simulink model "Cardiovascularmodel"  (Simulink 7.4)
settings: Solver=ode45  StartTime=0.0  StopTime=10.0  RelTol=1e-3
undefined symbols (not defined in the file): magnitude
(part 1 of 2)
settings Model: Creator=Marek  LastModifiedBy=Marek

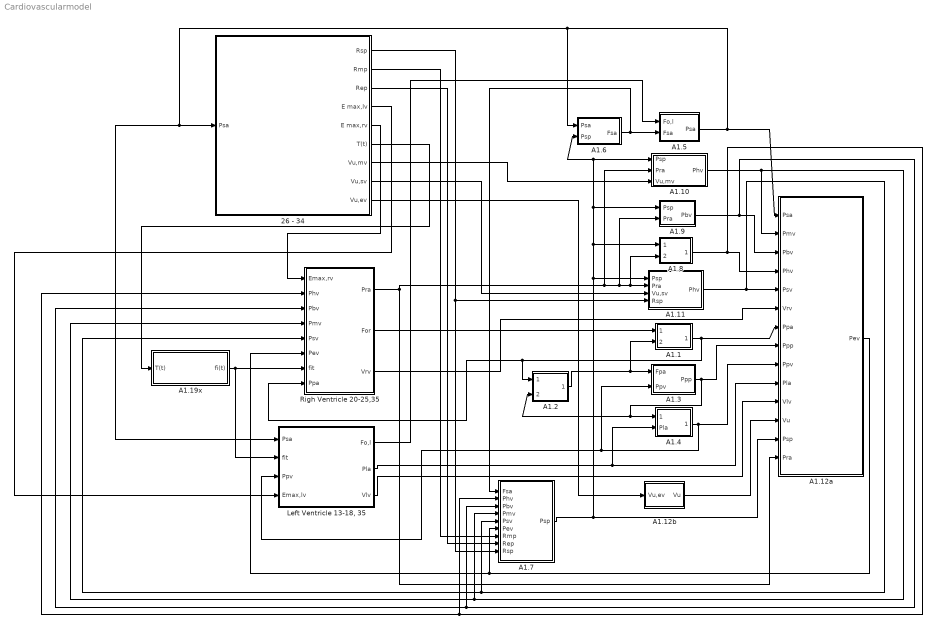
== system Cardiovascularmodel ==
  26 - 34 : Subsystem
  A1.1 : Subsystem
  A1.10 : Subsystem
  A1.11 : Subsystem
  A1.12a : Subsystem
  A1.12b : Subsystem
  A1.19x : Subsystem
  A1.2 : Subsystem
  A1.3 : Subsystem
  A1.4 : Subsystem
  A1.5 : Subsystem
  A1.6 : Subsystem
  A1.7 : Subsystem
  A1.8 : Subsystem
  A1.9 : Subsystem
  "Left Ventricle 13-18, 35" : Subsystem
  Righ Ventricle 20-25,35 : Subsystem
  wires:
  A1.11/1(Phv) -> A1.12a/5(Psv), A1.7/5(Psv), Righ Ventricle 20-25,35/5(Psv)
  A1.5/1(Psa) -> A1.12a/1(Psa), A1.6/1(Psa), 26 - 34/1(Psa), "Left Ventricle 13-18, 35"/1(Psa)
  A1.10/1(Phv) -> A1.12a/2(Pmv), A1.7/4(Pmv), Righ Ventricle 20-25,35/4(Pmv)
  A1.9/1(Pbv) -> A1.12a/3(Pbv), A1.7/3(Pbv), Righ Ventricle 20-25,35/3(Pbv)
  A1.8/1(Phv) -> A1.12a/4(Phv), A1.7/2(Phv), Righ Ventricle 20-25,35/2(Phv)
  Righ Ventricle 20-25,35/3(Vrv) -> A1.12a/6(Vrv)
  A1.1/1(Ppa) -> A1.12a/7(Ppa), A1.2/1(Ppa), Righ Ventricle 20-25,35/8(Ppa)
  A1.3/1(Ppp) -> A1.12a/8(Ppp), A1.2/2(Ppp), A1.4/1(Ppp)
  A1.4/1(Ppv) -> A1.12a/9(Ppv), A1.3/2(Ppv), "Left Ventricle 13-18, 35"/3(Ppv)
  "Left Ventricle 13-18, 35"/2(Pla) -> A1.12a/10(Pla), A1.4/2(Pla)
  A1.12b/1(Vu) -> A1.12a/12(Vu)
  A1.7/1(Psp) -> A1.12a/13(Psp), A1.8/1(Psp), A1.10/1(Psp), A1.6/2(Psp), A1.9/1(Psp), A1.11/1(Psp)
  A1.2/1(Fpa) -> A1.3/1(Fpa), A1.1/2(Fpa)
  Righ Ventricle 20-25,35/1(Pra) -> A1.12a/14(Pra), A1.11/2(Pra), A1.8/2(Pra), A1.9/2(Pra), A1.10/2(Pra)
  A1.6/1(Fsa) -> A1.5/2(Fsa), A1.7/1(Fsa)
  A1.19x/1(fi(t)) -> Righ Ventricle 20-25,35/7(fit), "Left Ventricle 13-18, 35"/2(fit)
  A1.12a/1(Pev) -> A1.7/6(Pev), Righ Ventricle 20-25,35/6(Pev)
  26 - 34/6(T(t)) -> A1.19x/1(T(t))
  "Left Ventricle 13-18, 35"/3(Vlv) -> A1.12a/11(Vlv)
  26 - 34/7(Vu,mv) -> A1.10/3(Vu,mv)
  26 - 34/8(Vu,sv) -> A1.11/3(Vu,sv)
  "Left Ventricle 13-18, 35"/1(Fo,l) -> A1.5/1(Fo,l)
  Righ Ventricle 20-25,35/2(For) -> A1.1/1(Fo,r)
  26 - 34/1(Rsp) -> A1.7/9(Rsp), A1.11/4(Rsp)
  26 - 34/2(Rmp) -> A1.7/7(Rmp)
  26 - 34/3(Rep) -> A1.7/8(Rep)
  26 - 34/9(Vu,ev) -> A1.12b/1(Vu,ev)
  26 - 34/5(E max,rv) -> Righ Ventricle 20-25,35/1(Emax,rv)
  26 - 34/4(E max,lv) -> "Left Ventricle 13-18, 35"/4(Emax,lv)

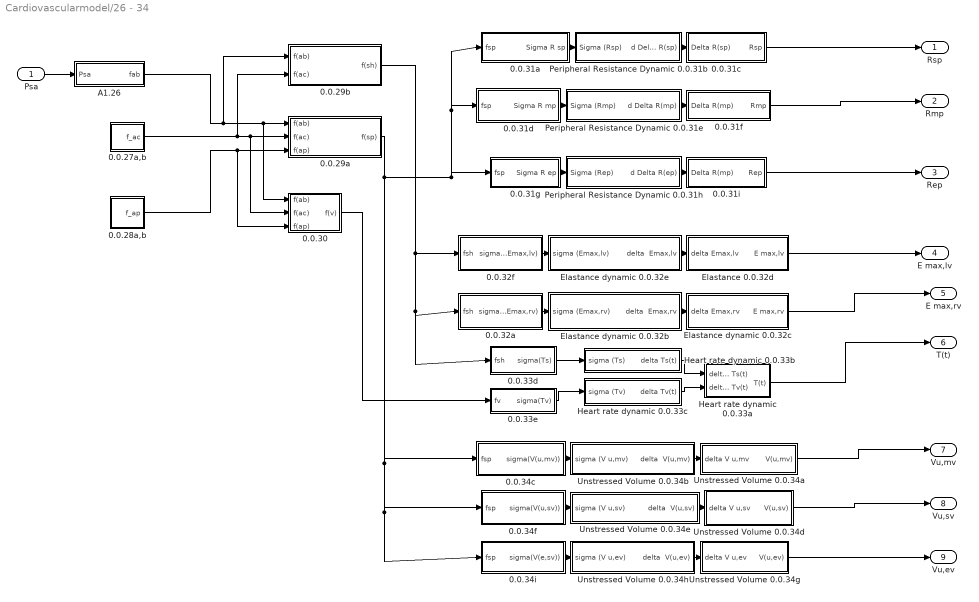
== system Cardiovascularmodel/26 - 34 ==
  Psa : Inport  OutDataType=fixdt(1, 16)  OutScaling=2^0
  0.0.27a,b : Subsystem
  0.0.28a,b : Subsystem
  0.0.29a : Subsystem
  0.0.29b : Subsystem
  0.0.30 : Subsystem
  0.0.31a : Subsystem
  0.0.31c : Subsystem
  0.0.31d : Subsystem
  0.0.31f : Subsystem
  0.0.31g : Subsystem
  0.0.31i : Subsystem
  0.0.32a : Subsystem
  0.0.32f : Subsystem
  0.0.33d : Subsystem
  0.0.33e : Subsystem
  0.0.34c : Subsystem
  0.0.34f : Subsystem
  0.0.34i : Subsystem
  A1.26 : Subsystem
  Elastance 0.0.32d : Subsystem
  Elastance dynamic 0.0.32b : Subsystem
  Elastance dynamic 0.0.32c : Subsystem
  Elastance dynamic 0.0.32e : Subsystem
  Heart rate dynamic 0.0.33a : Subsystem
  Heart rate dynamic 0.0.33b : Subsystem
  Heart rate dynamic 0.0.33c : Subsystem
  Peripheral Resistance Dynamic 0.0.31b : Subsystem
  Peripheral Resistance Dynamic 0.0.31e : Subsystem
  Peripheral Resistance Dynamic 0.0.31h : Subsystem
  Unstressed Volume 0.0.34a : Subsystem
  Unstressed Volume 0.0.34b : Subsystem
  Unstressed Volume 0.0.34d : Subsystem
  Unstressed Volume 0.0.34e : Subsystem
  Unstressed Volume 0.0.34g : Subsystem
  Unstressed Volume 0.0.34h : Subsystem
  Rsp : Outport  OutDataType=fixdt(1, 16)  OutScaling=2^0
  Rmp : Outport  Port=2  OutDataType=fixdt(1, 16)  OutScaling=2^0
  Rep : Outport  Port=3  OutDataType=fixdt(1, 16)  OutScaling=2^0
  E max,lv : Outport  Port=4  OutDataType=fixdt(1, 16)  OutScaling=2^0
  E max,rv : Outport  Port=5  OutDataType=fixdt(1, 16)  OutScaling=2^0
  T(t) : Outport  Port=6  OutDataType=fixdt(1, 16)  OutScaling=2^0
  Vu,mv : Outport  Port=7  OutDataType=fixdt(1, 16)  OutScaling=2^0
  Vu,sv : Outport  Port=8  OutDataType=fixdt(1, 16)  OutScaling=2^0
  Vu,ev : Outport  Port=9  OutDataType=fixdt(1, 16)  OutScaling=2^0
  wires:
  A1.26/1(fab) -> 0.0.29a/1(f(ab)), 0.0.30/1(f(ab)), 0.0.29b/1(f(ab))
  0.0.27a,b/1(f_ac) -> 0.0.29a/2(f(ac)), 0.0.30/2(f(ac)), 0.0.29b/2(f(ac))
  0.0.28a,b/1(f_ap) -> 0.0.29a/3(f(ap)), 0.0.30/3(f(ap))
  Elastance dynamic 0.0.32e/1(delta  Emax,lv) -> Elastance 0.0.32d/1(delta Emax,lv)
  0.0.32f/1(sigma(Emax,lv)) -> Elastance dynamic 0.0.32e/1(sigma (Emax,lv))
  Elastance dynamic 0.0.32b/1(delta  Emax,rv) -> Elastance dynamic 0.0.32c/1(delta Emax,rv)
  0.0.32a/1(sigma(Emax,rv)) -> Elastance dynamic 0.0.32b/1(sigma (Emax,rv))
  Heart rate dynamic 0.0.33c/1(delta Tv(t)) -> Heart rate dynamic 0.0.33a/2(delta Tv(t))
  0.0.33d/1(sigma(Ts)) -> Heart rate dynamic 0.0.33b/1(sigma (Ts))
  0.0.33e/1(sigma(Tv)) -> Heart rate dynamic 0.0.33c/1(sigma (Tv))
  Heart rate dynamic 0.0.33b/1(delta Ts(t)) -> Heart rate dynamic 0.0.33a/1(delta Ts(t))
  Unstressed Volume 0.0.34b/1(delta  V(u,mv)) -> Unstressed Volume 0.0.34a/1(delta V u,mv)
  0.0.34c/1(sigma(V(u,mv))) -> Unstressed Volume 0.0.34b/1(sigma (V u,mv))
  Unstressed Volume 0.0.34e/1(delta  V(u,sv)) -> Unstressed Volume 0.0.34d/1(delta V u,sv)
  0.0.34f/1(sigma(V(u,sv))) -> Unstressed Volume 0.0.34e/1(sigma (V u,sv))
  Unstressed Volume 0.0.34h/1(delta  V(u,ev)) -> Unstressed Volume 0.0.34g/1(delta V u,ev)
  0.0.34i/1(sigma(V(e,sv))) -> Unstressed Volume 0.0.34h/1(sigma (V u,ev))
  0.0.31a/1(Sigma R sp) -> Peripheral Resistance Dynamic 0.0.31b/1(Sigma (Rsp))
  Peripheral Resistance Dynamic 0.0.31b/1(d Delta R(sp)) -> 0.0.31c/1(Delta R(sp))
  0.0.31d/1(Sigma R mp) -> Peripheral Resistance Dynamic 0.0.31e/1(Sigma (Rmp))
  Peripheral Resistance Dynamic 0.0.31e/1(d Delta R(mp)) -> 0.0.31f/1(Delta R(mp))
  0.0.31g/1(Sigma R ep) -> Peripheral Resistance Dynamic 0.0.31h/1(Sigma (Rep))
  Peripheral Resistance Dynamic 0.0.31h/1(d Delta R(ep)) -> 0.0.31i/1(Delta R(mp))
  Psa/1 -> A1.26/1(Psa)
  0.0.29b/1(f(sh)) -> 0.0.32f/1(fsh), 0.0.32a/1(fsh), 0.0.33d/1(fsh)
  0.0.29a/1(f(sp)) -> 0.0.34i/1(fsp), 0.0.34f/1(fsp), 0.0.34c/1(fsp), 0.0.31g/1(fsp), 0.0.31d/1(fsp), 0.0.31a/1(fsp)
  0.0.30/1(f(v)) -> 0.0.33e/1(fv)
  0.0.31c/1(Rsp) -> Rsp/1
  0.0.31f/1(Rmp) -> Rmp/1
  0.0.31i/1(Rep) -> Rep/1
  Elastance 0.0.32d/1(E max,lv) -> E max,lv/1
  Elastance dynamic 0.0.32c/1(E max,rv) -> E max,rv/1
  Heart rate dynamic 0.0.33a/1(T(t)) -> T(t)/1
  Unstressed Volume 0.0.34a/1(V(u,mv)) -> Vu,mv/1
  Unstressed Volume 0.0.34d/1(V(u,sv)) -> Vu,sv/1
  Unstressed Volume 0.0.34g/1(V(u,ev)) -> Vu,ev/1

== system Cardiovascularmodel/A1.1 ==
  note: Ppa
  Fo,r : Inport  OutDataType=sfix(16)  OutScaling=2^0
  Fpa : Inport  Port=2  OutDataType=sfix(16)  OutScaling=2^0
  Constant : Constant  OutDataType=sfix(16)  OutScaling=2^0
  Cpa : Constant  Value=19.23  OutDataType=sfix(16)  OutScaling=2^0
  Divide : Product  Inputs=*/  OutDataType=sfix(16)  OutScaling=2^-10
  Integrator : Integrator
  Product : Product  OutDataType=sfix(16)  OutScaling=2^0  RndMeth=Zero
  Subtract : Sum  Inputs=+-  OutDataType=sfix(16)  OutScaling=2^-10
  Ppa : Outport  OutDataType=sfix(16)  OutScaling=2^0
  wires:
  Integrator/1 -> Ppa/1
  Constant/1 -> Divide/1
  Cpa/1 -> Divide/2
  Fo,r/1 -> Subtract/1
  Fpa/1 -> Subtract/2
  Product/1 -> Integrator/1
  Divide/1 -> Product/1
  Subtract/1 -> Product/2

== system Cardiovascularmodel/A1.10 ==
  note: Pmv
  Psp : Inport  OutDataType=sfix(16)  OutScaling=2^0
  Pra : Inport  Port=2  OutDataType=sfix(16)  OutScaling=2^0
  Vu,mv : Inport  Port=3  OutDataType=sfix(16)  OutScaling=2^0
  Cmv : Constant  Value=15.71  OutDataType=sfix(16)  OutScaling=2^0
  Constant : Constant  OutDataType=sfix(16)  OutScaling=2^0
  Derivative : Derivative
  Divide : Product  Inputs=*/  OutDataType=sfix(16)  OutScaling=2^-10
  Divide1 : Product  Inputs=*/  OutDataType=sfix(16)  OutScaling=2^-10
  Divide2 : Product  Inputs=*/  OutDataType=sfix(16)  OutScaling=2^-10
  Integrator : Integrator
  Product : Product  OutDataType=sfix(16)  OutScaling=2^0  RndMeth=Zero
  Rmp : Constant  Value=4.48  OutDataType=sfix(16)  OutScaling=2^0
  Rmv : Constant  Value=0.05  OutDataType=sfix(16)  OutScaling=2^0
  Subtract : Sum  Inputs=+-  OutDataType=sfix(16)  OutScaling=2^-10
  Subtract1 : Sum  Inputs=+-  OutDataType=sfix(16)  OutScaling=2^-10
  Sum : Sum  Inputs=+--  OutDataType=sfix(16)  OutScaling=2^0
  Phv : Outport  OutDataType=sfix(16)  OutScaling=2^0
  wires:
  Constant/1 -> Divide/1
  Cmv/1 -> Divide/2
  Divide/1 -> Product/1
  Psp/1 -> Subtract/1
  Pra/1 -> Subtract1/2
  Subtract/1 -> Divide1/1
  Rmp/1 -> Divide1/2
  Subtract1/1 -> Divide2/1
  Rmv/1 -> Divide2/2
  Divide1/1 -> Sum/1
  Divide2/1 -> Sum/2
  Sum/1 -> Product/2
  Product/1 -> Integrator/1
  Integrator/1 -> Phv/1, Subtract/2, Subtract1/1  "Pmv"
  Vu,mv/1 -> Derivative/1
  Derivative/1 -> Sum/3

== system Cardiovascularmodel/A1.11 ==
  note: Psv
  Psp : Inport  OutDataType=sfix(16)  OutScaling=2^0
  Pra : Inport  Port=2  OutDataType=sfix(16)  OutScaling=2^0
  Vu,sv : Inport  Port=3  OutDataType=sfix(16)  OutScaling=2^0
  Rsp : Inport  Port=4  OutDataType=sfix(16)  OutScaling=2^0
  Constant : Constant  OutDataType=sfix(16)  OutScaling=2^0
  Csv : Constant  Value=61.11  OutDataType=sfix(16)  OutScaling=2^0
  Derivative : Derivative
  Divide : Product  Inputs=*/  OutDataType=sfix(16)  OutScaling=2^-10
  Divide1 : Product  Inputs=*/  OutDataType=sfix(16)  OutScaling=2^-10
  Divide2 : Product  Inputs=*/  OutDataType=sfix(16)  OutScaling=2^-10
  Integrator : Integrator
  Product : Product  OutDataType=sfix(16)  OutScaling=2^0  RndMeth=Zero
  Rsv : Constant  Value=0.038  OutDataType=sfix(16)  OutScaling=2^0
  Subtract : Sum  Inputs=+-  OutDataType=sfix(16)  OutScaling=2^-10
  Subtract1 : Sum  Inputs=+-  OutDataType=sfix(16)  OutScaling=2^-10
  Sum : Sum  Inputs=+--  OutDataType=sfix(16)  OutScaling=2^0
  Phv : Outport  OutDataType=sfix(16)  OutScaling=2^0
  wires:
  Constant/1 -> Divide/1
  Csv/1 -> Divide/2
  Divide/1 -> Product/1
  Psp/1 -> Subtract/1
  Pra/1 -> Subtract1/2
  Subtract/1 -> Divide1/1
  Rsp/1 -> Divide1/2
  Subtract1/1 -> Divide2/1
  Rsv/1 -> Divide2/2
  Divide1/1 -> Sum/1
  Divide2/1 -> Sum/2
  Sum/1 -> Product/2
  Product/1 -> Integrator/1
  Integrator/1 -> Phv/1, Subtract/2, Subtract1/1  "Psv"
  Vu,sv/1 -> Derivative/1
  Derivative/1 -> Sum/3

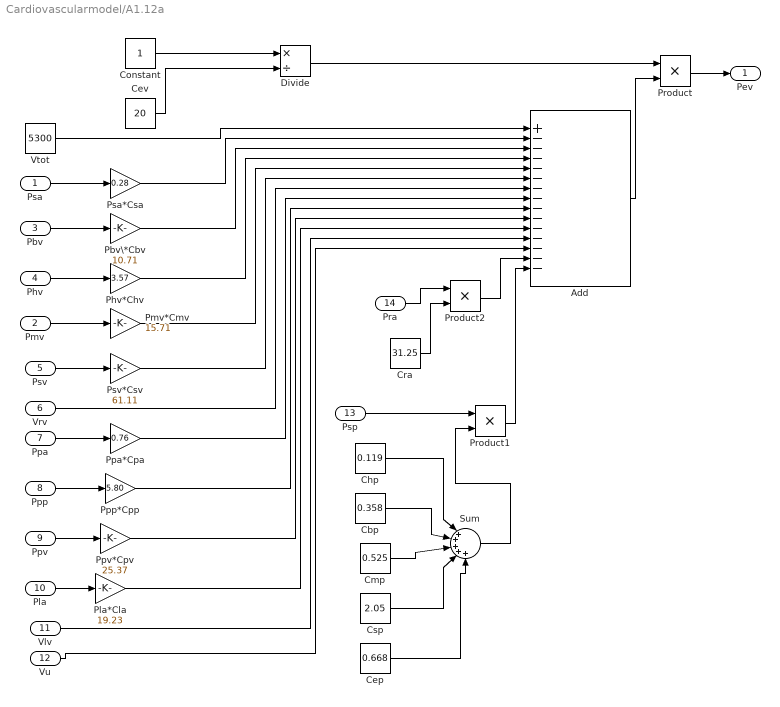
== system Cardiovascularmodel/A1.12a ==
  Psa : Inport  OutDataType=sfix(16)  OutScaling=2^0
  Pmv : Inport  Port=2  OutDataType=sfix(16)  OutScaling=2^0
  Pbv : Inport  Port=3  OutDataType=sfix(16)  OutScaling=2^0
  Phv : Inport  Port=4  OutDataType=sfix(16)  OutScaling=2^0
  Psv : Inport  Port=5  OutDataType=sfix(16)  OutScaling=2^0
  Vrv : Inport  Port=6  OutDataType=sfix(16)  OutScaling=2^0
  Ppa : Inport  Port=7  OutDataType=sfix(16)  OutScaling=2^0
  Ppp : Inport  Port=8  OutDataType=sfix(16)  OutScaling=2^0
  Ppv : Inport  Port=9  OutDataType=sfix(16)  OutScaling=2^0
  Pla : Inport  Port=10  OutDataType=sfix(16)  OutScaling=2^0
  Vlv : Inport  Port=11  OutDataType=sfix(16)  OutScaling=2^0
  Vu : Inport  Port=12  OutDataType=sfix(16)  OutScaling=2^0
  Psp : Inport  Port=13  OutDataType=sfix(16)  OutScaling=2^0
  Pra : Inport  Port=14  OutDataType=fixdt(1, 16)  OutScaling=2^0
  Add : Sum  Inputs=+--------------  OutDataType=sfix(16)  OutScaling=2^-10
  Cbp : Constant  Value=0.358  OutDataType=sfix(16)  OutScaling=2^0
  Cep : Constant  Value=0.668  OutDataType=sfix(16)  OutScaling=2^0
  Cev : Constant  Value=20  OutDataType=sfix(16)  OutScaling=2^0
  Chp : Constant  Value=0.119  OutDataType=sfix(16)  OutScaling=2^0
  Cmp : Constant  Value=0.525  OutDataType=sfix(16)  OutScaling=2^0
  Constant : Constant  OutDataType=sfix(16)  OutScaling=2^0
  Cra : Constant  Value=31.25  OutDataType=sfix(16)  OutScaling=2^0
  Csp : Constant  Value=2.05  OutDataType=sfix(16)  OutScaling=2^0
  Divide : Product  Inputs=*/  OutDataType=sfix(16)  OutScaling=2^-10
  Pbv\*Cbv : Gain  Gain=10.71  ParameterDataType=sfix(16)  ParameterScaling=2^0  OutDataType=sfix(16)  OutScaling=2^0
  Phv*Chv : Gain  Gain=3.57  ParameterDataType=sfix(16)  ParameterScaling=2^0  OutDataType=sfix(16)  OutScaling=2^0
  Pla*Cla : Gain  Gain=19.23  ParameterDataType=sfix(16)  ParameterScaling=2^0  OutDataType=sfix(16)  OutScaling=2^0
  Pmv*Cmv : Gain  Gain=15.71  ParameterDataType=sfix(16)  ParameterScaling=2^0  OutDataType=sfix(16)  OutScaling=2^0
  Ppa*Cpa : Gain  Gain=0.76  ParameterDataType=sfix(16)  ParameterScaling=2^0  OutDataType=sfix(16)  OutScaling=2^0
  Ppp*Cpp : Gain  Gain=5.80  ParameterDataType=sfix(16)  ParameterScaling=2^0  OutDataType=sfix(16)  OutScaling=2^0
  Ppv*Cpv : Gain  Gain=25.37  ParameterDataType=sfix(16)  ParameterScaling=2^0  OutDataType=sfix(16)  OutScaling=2^0
  Product : Product  OutDataType=sfix(16)  OutScaling=2^0  RndMeth=Zero
  Product1 : Product  OutDataType=sfix(16)  OutScaling=2^0  RndMeth=Zero
  Product2 : Product  OutDataType=fixdt(1, 16)  OutScaling=2^0  RndMeth=Zero
  Psa*Csa : Gain  Gain=0.28  ParameterDataType=sfix(16)  ParameterScaling=2^0  OutDataType=sfix(16)  OutScaling=2^0
  Psv*Csv : Gain  Gain=61.11  ParameterDataType=sfix(16)  ParameterScaling=2^0  OutDataType=sfix(16)  OutScaling=2^0
  Sum : Sum  Inputs=|+++++  OutDataType=sfix(16)  OutScaling=2^0
  Vtot : Constant  Value=5300  OutDataType=sfix(16)  OutScaling=2^0
  Pev : Outport  OutDataType=sfix(16)  OutScaling=2^0
  wires:
  Product/1 -> Pev/1
  Cep/1 -> Sum/5
  Csp/1 -> Sum/4
  Cmp/1 -> Sum/3
  Cbp/1 -> Sum/2
  Chp/1 -> Sum/1
  Psp/1 -> Product1/1
  Product1/1 -> Add/15
  Vu/1 -> Add/13
  Vlv/1 -> Add/12
  Pla*Cla/1 -> Add/11
  Pla/1 -> Pla*Cla/1
  Ppv*Cpv/1 -> Add/10
  Ppv/1 -> Ppv*Cpv/1
  Ppp*Cpp/1 -> Add/9
  Ppp/1 -> Ppp*Cpp/1
  Ppa*Cpa/1 -> Add/8
  Ppa/1 -> Ppa*Cpa/1
  Vrv/1 -> Add/7
  Psv*Csv/1 -> Add/6
  Psv/1 -> Psv*Csv/1
  Pmv*Cmv/1 -> Add/5
  Pmv/1 -> Pmv*Cmv/1
  Phv*Chv/1 -> Add/4
  Phv/1 -> Phv*Chv/1
  Pbv\*Cbv/1 -> Add/3
  Pbv/1 -> Pbv\*Cbv/1
  Psa*Csa/1 -> Add/2
  Psa/1 -> Psa*Csa/1
  Add/1 -> Product/2
  Vtot/1 -> Add/1
  Divide/1 -> Product/1
  Cev/1 -> Divide/2
  Constant/1 -> Divide/1
  Sum/1 -> Product1/2
  Pra/1 -> Product2/1
  Cra/1 -> Product2/2
  Product2/1 -> Add/14

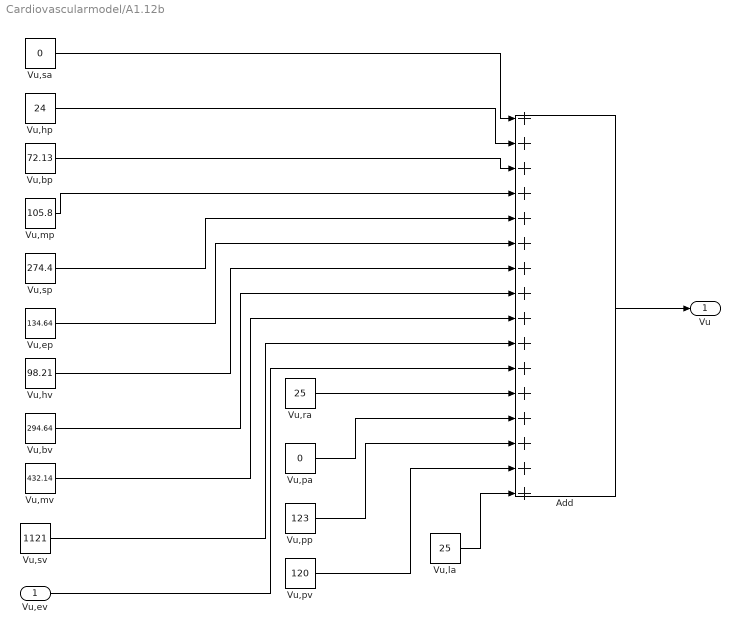
== system Cardiovascularmodel/A1.12b ==
  Vu,ev : Inport  OutDataType=fixdt(1, 16)  OutScaling=2^0
  Add : Sum  Inputs=++++++++++++++++  OutDataType=sfix(16)  OutScaling=2^-10
  Vu,bp : Constant  Value=72.13  OutDataType=sfix(16)  OutScaling=2^0
  Vu,bv : Constant  Value=294.64  OutDataType=sfix(16)  OutScaling=2^0
  Vu,ep : Constant  Value=134.64  OutDataType=sfix(16)  OutScaling=2^0
  Vu,hp : Constant  Value=24  OutDataType=sfix(16)  OutScaling=2^0
  Vu,hv : Constant  Value=98.21  OutDataType=sfix(16)  OutScaling=2^0
  Vu,la : Constant  Value=25  OutDataType=sfix(16)  OutScaling=2^0
  Vu,mp : Constant  Value=105.8  OutDataType=sfix(16)  OutScaling=2^0
  Vu,mv : Constant  Value=432.14  OutDataType=sfix(16)  OutScaling=2^0
  Vu,pa : Constant  Value=0  OutDataType=sfix(16)  OutScaling=2^0
  Vu,pp : Constant  Value=123  OutDataType=sfix(16)  OutScaling=2^0
  Vu,pv : Constant  Value=120  OutDataType=sfix(16)  OutScaling=2^0
  Vu,ra : Constant  Value=25  OutDataType=sfix(16)  OutScaling=2^0
  Vu,sa : Constant  Value=0  OutDataType=sfix(16)  OutScaling=2^0
  Vu,sp : Constant  Value=274.4  OutDataType=sfix(16)  OutScaling=2^0
  Vu,sv : Constant  Value=1121  OutDataType=sfix(16)  OutScaling=2^0
  Vu : Outport  OutDataType=sfix(16)  OutScaling=2^0
  wires:
  Add/1 -> Vu/1
  Vu,la/1 -> Add/16
  Vu,pv/1 -> Add/15
  Vu,pp/1 -> Add/14
  Vu,pa/1 -> Add/13
  Vu,ra/1 -> Add/12
  Vu,ev/1 -> Add/11
  Vu,sv/1 -> Add/10
  Vu,mv/1 -> Add/9
  Vu,bv/1 -> Add/8
  Vu,hv/1 -> Add/7
  Vu,ep/1 -> Add/6
  Vu,sp/1 -> Add/5
  Vu,mp/1 -> Add/4
  Vu,bp/1 -> Add/3
  Vu,hp/1 -> Add/2
  Vu,sa/1 -> Add/1

== system Cardiovascularmodel/A1.19x ==
  T(t) : Inport  OutDataType=sfix(16)  OutScaling=2^0
  A1.19 : Subsystem
  A1.19a : Subsystem
  A1.19b : Subsystem
  A1.19c : Subsystem
  fi(t) : Outport  OutDataType=sfix(16)  OutScaling=2^0
  wires:
  A1.19b/1(ksi) -> A1.19a/1(ksi)
  A1.19a/1(u(t)) -> A1.19/3(u(t))
  A1.19c/1(T,sys) -> A1.19/1(T,sys)
  T(t)/1 -> A1.19/2(T(t)), A1.19b/1(T(t))
  A1.19/1(fi(t)) -> fi(t)/1

== system Cardiovascularmodel/A1.2 ==
  note: Ppa
  Ppa : Inport  OutDataType=sfix(16)  OutScaling=2^0
  Ppp : Inport  Port=2  OutDataType=sfix(16)  OutScaling=2^0
  Constant : Constant  OutDataType=sfix(16)  OutScaling=2^0
  Divide : Product  Inputs=*/  OutDataType=sfix(16)  OutScaling=2^-10
  Integrator : Integrator
  Lpa : Constant  Value=0.18*1E-3  OutDataType=sfix(16)  OutScaling=2^0
  Product : Product  OutDataType=sfix(16)  OutScaling=2^0  RndMeth=Zero
  Rpa*Fpa : Gain  Gain=0.023  ParameterDataType=sfix(16)  ParameterScaling=2^0  OutDataType=sfix(16)  OutScaling=2^0
  Sum : Sum  Inputs=+--  OutDataType=sfix(16)  OutScaling=2^0
  Fpa : Outport  OutDataType=sfix(16)  OutScaling=2^0
  wires:
  Constant/1 -> Divide/1
  Lpa/1 -> Divide/2
  Divide/1 -> Product/1
  Ppa/1 -> Sum/1
  Ppp/1 -> Sum/2
  Integrator/1 -> Rpa*Fpa/1, Fpa/1  "Fpa"
  Rpa*Fpa/1 -> Sum/3
  Sum/1 -> Product/2
  Product/1 -> Integrator/1  "dFpa/dt"

== system Cardiovascularmodel/A1.3 ==
  Fpa : Inport  OutDataType=sfix(16)  OutScaling=2^0
  Ppv : Inport  Port=2  OutDataType=sfix(16)  OutScaling=2^0
  ((Ppp-Ppv)/Rpp)*(1/Cpp) : Product  OutDataType=sfix(16)  OutScaling=2^0  RndMeth=Zero
  Constant : Constant  OutDataType=sfix(16)  OutScaling=2^0
  Cpp : Constant  Value=5.80  OutDataType=sfix(16)  OutScaling=2^0
  Divide : Product  Inputs=*/  OutDataType=sfix(16)  OutScaling=2^-10
  Divide1 : Product  Inputs=*/  OutDataType=sfix(16)  OutScaling=2^-10
  Fpa*(1/Cpp) : Product  OutDataType=sfix(16)  OutScaling=2^0  RndMeth=Zero
  Integrator : Integrator
  Rpp : Constant  Value=0.0894  OutDataType=sfix(16)  OutScaling=2^0
  Subtract : Sum  Inputs=+-  OutDataType=sfix(16)  OutScaling=2^-10
  Subtract1 : Sum  Inputs=+-  OutDataType=sfix(16)  OutScaling=2^-10
  Ppp : Outport  OutDataType=sfix(16)  OutScaling=2^0
  wires:
  Constant/1 -> Divide/1
  Cpp/1 -> Divide/2
  Divide/1 -> Fpa*(1/Cpp)/1, ((Ppp-Ppv)/Rpp)*(1/Cpp)/1
  Ppv/1 -> Subtract/2
  Subtract/1 -> Divide1/1
  Rpp/1 -> Divide1/2
  Fpa*(1/Cpp)/1 -> Subtract1/1
  Subtract1/1 -> Integrator/1
  Integrator/1 -> Ppp/1, Subtract/1
  Fpa/1 -> Fpa*(1/Cpp)/2
  Divide1/1 -> ((Ppp-Ppv)/Rpp)*(1/Cpp)/2
  ((Ppp-Ppv)/Rpp)*(1/Cpp)/1 -> Subtract1/2

== system Cardiovascularmodel/A1.4 ==
  Ppp : Inport  OutDataType=sfix(16)  OutScaling=2^0
  Pla : Inport  Port=2  OutDataType=sfix(16)  OutScaling=2^0
  Constant : Constant  OutDataType=sfix(16)  OutScaling=2^0
  Cpv : Constant  Value=25.37  OutDataType=sfix(16)  OutScaling=2^0
  Divide : Product  Inputs=*/  OutDataType=sfix(16)  OutScaling=2^-10
  Divide1 : Product  Inputs=*/  OutDataType=sfix(16)  OutScaling=2^-10
  Divide2 : Product  Inputs=*/  OutDataType=sfix(16)  OutScaling=2^-10
  Integrator : Integrator
  Product : Product  OutDataType=sfix(16)  OutScaling=2^0  RndMeth=Zero
  Rpp : Constant  Value=0.0894  OutDataType=sfix(16)  OutScaling=2^0
  Rpv : Constant  Value=0.0056  OutDataType=sfix(16)  OutScaling=2^0
  Subtract : Sum  Inputs=+-  OutDataType=sfix(16)  OutScaling=2^-10
  Subtract1 : Sum  Inputs=+-  OutDataType=sfix(16)  OutScaling=2^-10
  Subtract2 : Sum  Inputs=+-  OutDataType=sfix(16)  OutScaling=2^-10
  Ppv : Outport  OutDataType=sfix(16)  OutScaling=2^0
  wires:
  Constant/1 -> Divide/1
  Cpv/1 -> Divide/2
  Divide/1 -> Product/1
  Ppp/1 -> Subtract/1
  Pla/1 -> Subtract1/2
  Subtract/1 -> Divide1/1
  Rpp/1 -> Divide1/2
  Subtract1/1 -> Divide2/1
  Rpv/1 -> Divide2/2
  Divide1/1 -> Subtract2/1
  Divide2/1 -> Subtract2/2
  Subtract2/1 -> Product/2
  Product/1 -> Integrator/1
  Integrator/1 -> Ppv/1, Subtract/2, Subtract1/1  "Ppv"

== system Cardiovascularmodel/A1.5 ==
  note: Psa
  Fo,l : Inport  OutDataType=sfix(16)  OutScaling=2^0
  Fsa : Inport  Port=2  OutDataType=sfix(16)  OutScaling=2^0
  Constant : Constant  OutDataType=sfix(16)  OutScaling=2^0
  Csa : Constant  Value=0.28  OutDataType=sfix(16)  OutScaling=2^0
  Divide : Product  Inputs=*/  OutDataType=sfix(16)  OutScaling=2^-10
  Integrator : Integrator
  Product : Product  OutDataType=sfix(16)  OutScaling=2^0  RndMeth=Zero
  Subtract : Sum  Inputs=+-  OutDataType=sfix(16)  OutScaling=2^-10
  Psa : Outport  OutDataType=sfix(16)  OutScaling=2^0
  wires:
  Integrator/1 -> Psa/1
  Constant/1 -> Divide/1
  Csa/1 -> Divide/2
  Fo,l/1 -> Subtract/1
  Fsa/1 -> Subtract/2
  Product/1 -> Integrator/1
  Divide/1 -> Product/1
  Subtract/1 -> Product/2

== system Cardiovascularmodel/A1.6 ==
  note: Psa
  Psa : Inport  OutDataType=sfix(16)  OutScaling=2^0
  Psp : Inport  Port=2  OutDataType=sfix(16)  OutScaling=2^0
  Constant : Constant  OutDataType=sfix(16)  OutScaling=2^0
  Divide : Product  Inputs=*/  OutDataType=sfix(16)  OutScaling=2^-10
  Integrator : Integrator
  Lsa : Constant  Value=0.00022  OutDataType=sfix(16)  OutScaling=2^0
  Product : Product  OutDataType=sfix(16)  OutScaling=2^0  RndMeth=Zero
  Product1 : Product  OutDataType=sfix(16)  OutScaling=2^0  RndMeth=Zero
  Rsa : Constant  Value=0.06  OutDataType=sfix(16)  OutScaling=2^0
  Sum : Sum  Inputs=+--  OutDataType=sfix(16)  OutScaling=2^0
  Fsa : Outport  OutDataType=sfix(16)  OutScaling=2^0
  wires:
  Constant/1 -> Divide/1
  Lsa/1 -> Divide/2
  Divide/1 -> Product/1
  Psa/1 -> Sum/1
  Psp/1 -> Sum/3
  Product/1 -> Integrator/1  "dFsa/dt"
  Sum/1 -> Product/2
  Integrator/1 -> Product1/2, Fsa/1  "Fsa"
  Product1/1 -> Sum/2
  Rsa/1 -> Product1/1

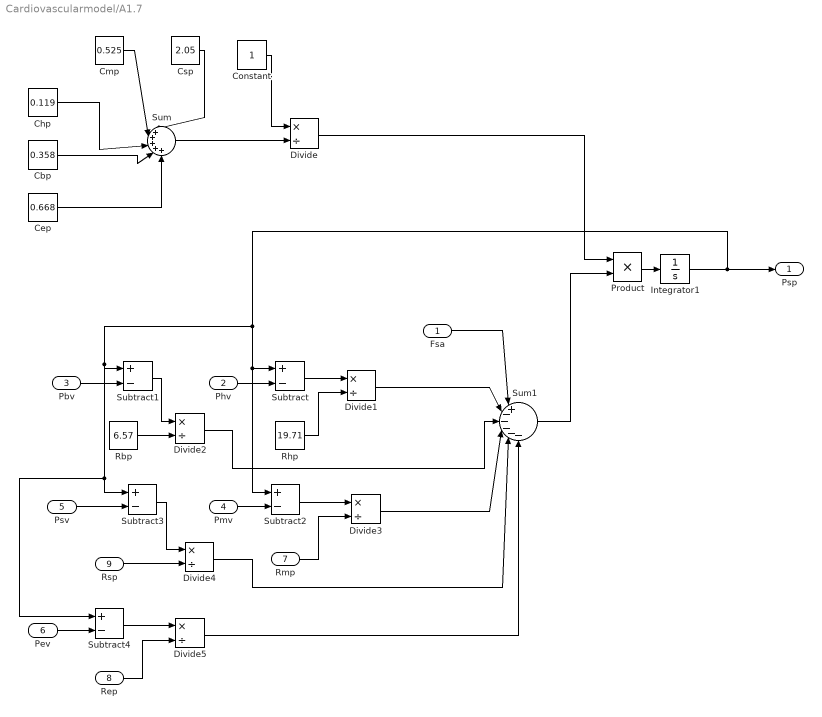
== system Cardiovascularmodel/A1.7 ==
  Fsa : Inport  OutDataType=sfix(16)  OutScaling=2^0
  Phv : Inport  Port=2  OutDataType=sfix(16)  OutScaling=2^0
  Pbv : Inport  Port=3  OutDataType=sfix(16)  OutScaling=2^0
  Pmv : Inport  Port=4  OutDataType=sfix(16)  OutScaling=2^0
  Psv : Inport  Port=5  OutDataType=sfix(16)  OutScaling=2^0
  Pev : Inport  Port=6  OutDataType=sfix(16)  OutScaling=2^0
  Rmp : Inport  Port=7  OutDataType=sfix(16)  OutScaling=2^0
  Rep : Inport  Port=8  OutDataType=sfix(16)  OutScaling=2^0
  Rsp : Inport  Port=9  OutDataType=sfix(16)  OutScaling=2^0
  Cbp : Constant  Value=0.358  OutDataType=sfix(16)  OutScaling=2^0
  Cep : Constant  Value=0.668  OutDataType=sfix(16)  OutScaling=2^0
  Chp : Constant  Value=0.119  OutDataType=sfix(16)  OutScaling=2^0
  Cmp : Constant  Value=0.525  OutDataType=sfix(16)  OutScaling=2^0
  Constant : Constant  OutDataType=sfix(16)  OutScaling=2^0
  Csp : Constant  Value=2.05  OutDataType=sfix(16)  OutScaling=2^0
  Divide{,1..5} (6 alike) : Product  Inputs=*/  OutDataType=sfix(16)  OutScaling=2^-10
  Integrator1 : Integrator
  Product : Product  OutDataType=sfix(16)  OutScaling=2^0  RndMeth=Zero
  Rbp : Constant  Value=6.57  OutDataType=sfix(16)  OutScaling=2^0
  Rhp : Constant  Value=19.71  OutDataType=sfix(16)  OutScaling=2^0
  Subtract{,1..4} (5 alike) : Sum  Inputs=+-  OutDataType=sfix(16)  OutScaling=2^-10
  Sum : Sum  Inputs=|+++++  OutDataType=sfix(16)  OutScaling=2^0
  Sum1 : Sum  Inputs=|+-----  OutDataType=sfix(16)  OutScaling=2^0
  Psp : Outport  OutDataType=sfix(16)  OutScaling=2^0
  wires:
  Cep/1 -> Sum/5
  Cbp/1 -> Sum/4
  Chp/1 -> Sum/3
  Cmp/1 -> Sum/2
  Csp/1 -> Sum/1
  Sum/1 -> Divide/2
  Constant/1 -> Divide/1
  Phv/1 -> Subtract/2
  Subtract/1 -> Divide1/1
  Rhp/1 -> Divide1/2
  Pbv/1 -> Subtract1/2
  Subtract1/1 -> Divide2/1
  Rbp/1 -> Divide2/2
  Pmv/1 -> Subtract2/2
  Subtract2/1 -> Divide3/1
  Rmp/1 -> Divide3/2
  Psv/1 -> Subtract3/2
  Subtract3/1 -> Divide4/1
  Rsp/1 -> Divide4/2
  Pev/1 -> Subtract4/2
  Subtract4/1 -> Divide5/1
  Rep/1 -> Divide5/2
  Fsa/1 -> Sum1/1
  Divide1/1 -> Sum1/2
  Divide2/1 -> Sum1/3
  Divide3/1 -> Sum1/4
  Divide4/1 -> Sum1/5
  Divide5/1 -> Sum1/6
  Divide/1 -> Product/1
  Sum1/1 -> Product/2
  Product/1 -> Integrator1/1
  Integrator1/1 -> Psp/1, Subtract/1, Subtract2/1, Subtract1/1, Subtract3/1, Subtract4/1

== system Cardiovascularmodel/A1.8 ==
  Psp : Inport  OutDataType=sfix(16)  OutScaling=2^0
  Pra : Inport  Port=2  OutDataType=sfix(16)  OutScaling=2^0
  Chv : Constant  Value=3.57  OutDataType=sfix(16)  OutScaling=2^0
  Constant : Constant  OutDataType=sfix(16)  OutScaling=2^0
  Divide : Product  Inputs=*/  OutDataType=sfix(16)  OutScaling=2^-10
  Divide1 : Product  Inputs=*/  OutDataType=sfix(16)  OutScaling=2^-10
  Divide2 : Product  Inputs=*/  OutDataType=sfix(16)  OutScaling=2^-10
  Integrator : Integrator
  Product : Product  OutDataType=sfix(16)  OutScaling=2^0  RndMeth=Zero
  Rhp : Constant  Value=19.71  OutDataType=sfix(16)  OutScaling=2^0
  Rhv : Constant  Value=0.224  OutDataType=sfix(16)  OutScaling=2^0
  Subtract : Sum  Inputs=+-  OutDataType=sfix(16)  OutScaling=2^-10
  Subtract1 : Sum  Inputs=+-  OutDataType=sfix(16)  OutScaling=2^-10
  Subtract2 : Sum  Inputs=+-  OutDataType=sfix(16)  OutScaling=2^-10
  Phv : Outport  OutDataType=sfix(16)  OutScaling=2^0
  wires:
  Constant/1 -> Divide/1
  Chv/1 -> Divide/2
  Divide/1 -> Product/1
  Psp/1 -> Subtract/1
  Pra/1 -> Subtract1/2
  Subtract/1 -> Divide1/1
  Rhp/1 -> Divide1/2
  Subtract1/1 -> Divide2/1
  Rhv/1 -> Divide2/2
  Divide1/1 -> Subtract2/1
  Divide2/1 -> Subtract2/2
  Subtract2/1 -> Product/2
  Product/1 -> Integrator/1
  Integrator/1 -> Phv/1, Subtract/2, Subtract1/1  "Phv"

== system Cardiovascularmodel/A1.9 ==
  Psp : Inport  OutDataType=sfix(16)  OutScaling=2^0
  Pra : Inport  Port=2  OutDataType=sfix(16)  OutScaling=2^0
  Cbv : Constant  Value=10.71  OutDataType=sfix(16)  OutScaling=2^0
  Constant : Constant  OutDataType=sfix(16)  OutScaling=2^0
  Divide : Product  Inputs=*/  OutDataType=sfix(16)  OutScaling=2^-10
  Divide1 : Product  Inputs=*/  OutDataType=sfix(16)  OutScaling=2^-10
  Divide2 : Product  Inputs=*/  OutDataType=sfix(16)  OutScaling=2^-10
  Integrator : Integrator
  Product : Product  OutDataType=sfix(16)  OutScaling=2^0  RndMeth=Zero
  Rbp : Constant  Value=6.57  OutDataType=sfix(16)  OutScaling=2^0
  Rbv : Constant  Value=0.075  OutDataType=sfix(16)  OutScaling=2^0
  Subtract : Sum  Inputs=+-  OutDataType=sfix(16)  OutScaling=2^-10
  Subtract1 : Sum  Inputs=+-  OutDataType=sfix(16)  OutScaling=2^-10
  Subtract2 : Sum  Inputs=+-  OutDataType=sfix(16)  OutScaling=2^-10
  Pbv : Outport  OutDataType=sfix(16)  OutScaling=2^0
  wires:
  Constant/1 -> Divide/1
  Cbv/1 -> Divide/2
  Divide/1 -> Product/1
  Psp/1 -> Subtract/1
  Pra/1 -> Subtract1/2
  Subtract/1 -> Divide1/1
  Rbp/1 -> Divide1/2
  Subtract1/1 -> Divide2/1
  Rbv/1 -> Divide2/2
  Divide1/1 -> Subtract2/1
  Divide2/1 -> Subtract2/2
  Subtract2/1 -> Product/2
  Product/1 -> Integrator/1
  Integrator/1 -> Pbv/1, Subtract/2, Subtract1/1  "Pbv"

== system Cardiovascularmodel/Left Ventricle 13-18, 35 ==
  Psa : Inport  OutDataType=fixdt(1, 16)  OutScaling=2^0
  fit : Inport  Port=2  OutDataType=fixdt(1, 16)  OutScaling=2^0
  Ppv : Inport  Port=3  OutDataType=fixdt(1, 16)  OutScaling=2^0
  Emax,lv : Inport  Port=4  OutDataType=sfix(16)  OutScaling=2^0
  0.0.35_Plv : Subsystem
  A1.13 : Subsystem
  A1.14 : Subsystem
  A1.15 : Subsystem
  A1.16 : Subsystem
  A1.17 : Subsystem
  A1.18 : Subsystem
  Fo,l : Outport  OutDataType=fixdt(1, 16)  OutScaling=2^0
  Pla : Outport  Port=2  OutDataType=fixdt(1, 16)  OutScaling=2^0
  Vlv : Outport  Port=3  OutDataType=fixdt(1, 16)  OutScaling=2^0
  wires:
  A1.18/1(P,max,lv(t)) -> A1.17/1(Pmax,lv), A1.16/2(Pmax,lv), 0.0.35_Plv/1(Pmax,lv)
  A1.15/1(Vlv) -> Vlv/1, A1.18/2(Vlv)
  A1.16/1(Fo,l) -> A1.15/2(Fo,l), 0.0.35_Plv/3(Fo,l), Fo,l/1
  A1.14/1(Fi,l) -> A1.15/1(Fi,l), A1.13/2(Fi,l)
  A1.17/1(Rlv) -> A1.16/3(Rlv), 0.0.35_Plv/2(Rl,v)
  A1.13/1(Pla) -> A1.14/2(Pla), Pla/1
  0.0.35_Plv/1(Plv) -> A1.14/1(Plv)
  Ppv/1 -> A1.13/1(Ppv)
  fit/1 -> A1.18/1(fi(t))
  Psa/1 -> A1.16/1(Psa)
  Emax,lv/1 -> A1.18/3(Emax,lv)

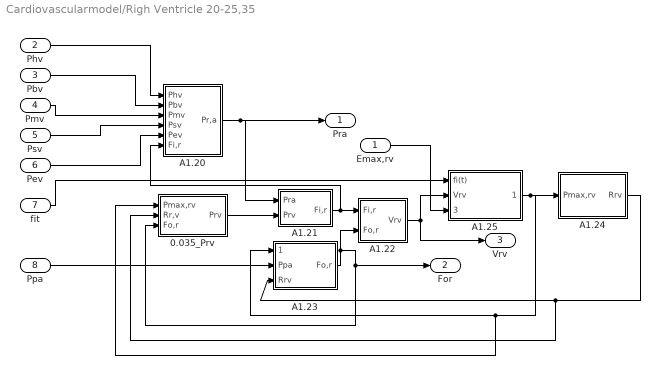
== system Cardiovascularmodel/Righ Ventricle 20-25,35 ==
  Emax,rv : Inport  OutDataType=sfix(16)  OutScaling=2^0
  Phv : Inport  Port=2  OutDataType=fixdt(1, 16)  OutScaling=2^0
  Pbv : Inport  Port=3  OutDataType=fixdt(1, 16)  OutScaling=2^0
  Pmv : Inport  Port=4  OutDataType=fixdt(1, 16)  OutScaling=2^0
  Psv : Inport  Port=5  OutDataType=fixdt(1, 16)  OutScaling=2^0
  Pev : Inport  Port=6  OutDataType=fixdt(1, 16)  OutScaling=2^0
  fit : Inport  Port=7  OutDataType=fixdt(1, 16)  OutScaling=2^0
  Ppa : Inport  Port=8  OutDataType=fixdt(1, 16)  OutScaling=2^0
  0.035_Prv : Subsystem
  A1.20 : Subsystem
  A1.21 : Subsystem
  A1.22 : Subsystem
  A1.23 : Subsystem
  A1.24 : Subsystem
  A1.25 : Subsystem
  Pra : Outport  OutDataType=fixdt(1, 16)  OutScaling=2^0
  For : Outport  Port=2  OutDataType=fixdt(1, 16)  OutScaling=2^0
  Vrv : Outport  Port=3  OutDataType=fixdt(1, 16)  OutScaling=2^0
  wires:
  A1.25/1(Pmax,rv(t)) -> A1.24/1(Pmax,rv), A1.23/1(Pmax,rv), 0.035_Prv/1(Pmax,rv)
  A1.22/1(Vrv) -> A1.25/2(Vrv), Vrv/1
  A1.23/1(Fo,r) -> A1.22/2(Fo,r), 0.035_Prv/3(Fo,r), For/1
  A1.21/1(Fi,r) -> A1.22/1(Fi,r), A1.20/6(Fi,r)
  A1.24/1(Rrv) -> A1.23/3(Rrv), 0.035_Prv/2(Rr,v)
  A1.20/1(Pr,a) -> A1.21/1(Pra), Pra/1
  0.035_Prv/1(Prv) -> A1.21/2(Prv)
  Ppa/1 -> A1.23/2(Ppa)
  fit/1 -> A1.25/1(fi(t))
  Pmv/1 -> A1.20/3(Pmv)
  Pbv/1 -> A1.20/2(Pbv)
  Phv/1 -> A1.20/1(Phv)
  Psv/1 -> A1.20/4(Psv)
  Pev/1 -> A1.20/5(Pev)
  Emax,rv/1 -> A1.25/3(Emax.rv)

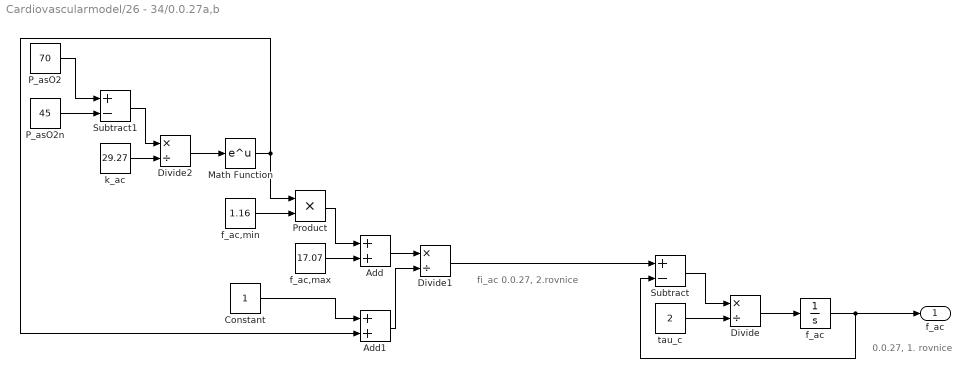
== system Cardiovascularmodel/26 - 34/0.0.27a,b ==
  note: fi_ac
      | 0.0.27, 2.rovnice
  note: 0.0.27, 1. rovnice
  Add : Sum  OutDataType=sfix(16)  OutScaling=2^-10
  Add1 : Sum  OutDataType=sfix(16)  OutScaling=2^-10
  Constant : Constant  OutDataType=sfix(16)  OutScaling=2^0
  Divide : Product  Inputs=*/  OutDataType=sfix(16)  OutScaling=2^-10
  Divide1 : Product  Inputs=*/  OutDataType=sfix(16)  OutScaling=2^-10
  Divide2 : Product  Inputs=*/  OutDataType=sfix(16)  OutScaling=2^-10
  Math Function : Math  OutDataType=sfix(16)  OutScaling=2^0  SaturateOnIntegerOverflow=on
  P_asO2 : Constant  Value=70  OutDataType=sfix(16)  OutScaling=2^0
  P_asO2n : Constant  Value=45  OutDataType=sfix(16)  OutScaling=2^0
  Product : Product  OutDataType=sfix(16)  OutScaling=2^0  RndMeth=Zero
  Subtract : Sum  Inputs=+-  OutDataType=sfix(16)  OutScaling=2^-10
  Subtract1 : Sum  Inputs=+-  OutDataType=sfix(16)  OutScaling=2^-10
  "f_ac  " : Integrator
  f_ac,max : Constant  Value=17.07  OutDataType=sfix(16)  OutScaling=2^0
  f_ac,min : Constant  Value=1.16  OutDataType=sfix(16)  OutScaling=2^0
  k_ac : Constant  Value=29.27  OutDataType=sfix(16)  OutScaling=2^0
  tau_c : Constant  Value=2  OutDataType=sfix(16)  OutScaling=2^0
  f_ac : Outport  OutDataType=sfix(16)  OutScaling=2^0
  wires:
  "f_ac  "/1 -> Subtract/2, f_ac/1
  Divide/1 -> "f_ac  "/1
  tau_c/1 -> Divide/2
  Subtract/1 -> Divide/1
  Add/1 -> Divide1/1
  f_ac,max/1 -> Add/2
  Product/1 -> Add/1
  f_ac,min/1 -> Product/2
  Math Function/1 -> Product/1, Add1/2
  Divide2/1 -> Math Function/1
  k_ac/1 -> Divide2/2
  Subtract1/1 -> Divide2/1
  P_asO2n/1 -> Subtract1/2
  P_asO2/1 -> Subtract1/1
  Add1/1 -> Divide1/2
  Constant/1 -> Add1/1
  Divide1/1 -> Subtract/1

== system Cardiovascularmodel/26 - 34/0.0.28a,b ==
  note: fi_ap
      | 0.0.28, 2.rovnice
  note: 0.0.28, 1.rovnice
  Divide : Product  Inputs=*/  OutDataType=sfix(16)  OutScaling=2^-10
  G_ap : Constant  Value=1/23291  OutDataType=sfix(16)  OutScaling=2^0
  Subtract : Sum  Inputs=+-  OutDataType=sfix(16)  OutScaling=2^-10
  V_T : Constant  Value=0.583  OutDataType=sfix(16)  OutScaling=2^0
  "f_ap " : Integrator
  fi_ap : Product  OutDataType=sfix(16)  OutScaling=2^0  RndMeth=Zero
  tau_p : Constant  Value=2  OutDataType=sfix(16)  OutScaling=2^0
  f_ap : Outport  OutDataType=sfix(16)  OutScaling=2^0
  wires:
  "f_ap "/1 -> Subtract/2, f_ap/1
  Divide/1 -> "f_ap "/1
  tau_p/1 -> Divide/2
  Subtract/1 -> Divide/1
  V_T/1 -> fi_ap/2
  G_ap/1 -> fi_ap/1
  fi_ap/1 -> Subtract/1

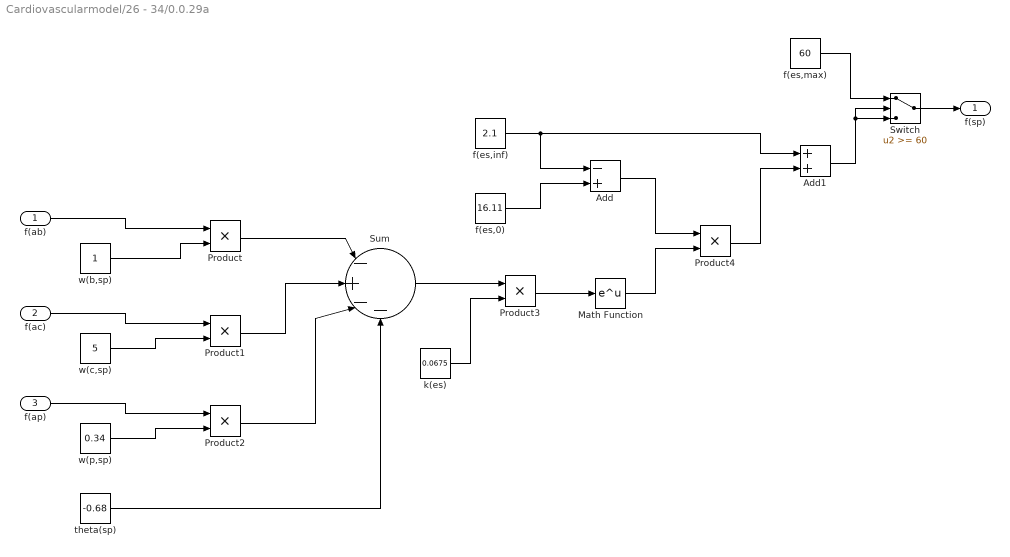
== system Cardiovascularmodel/26 - 34/0.0.29a ==
  f(ab) : Inport  OutDataType=sfix(16)  OutScaling=2^0
  f(ac) : Inport  Port=2  OutDataType=sfix(16)  OutScaling=2^0
  f(ap) : Inport  Port=3  OutDataType=sfix(16)  OutScaling=2^0
  Add : Sum  Inputs=-+  OutDataType=sfix(16)  OutScaling=2^-10
  Add1 : Sum  OutDataType=sfix(16)  OutScaling=2^-10
  Math Function : Math  OutDataType=sfix(16)  OutScaling=2^0  SaturateOnIntegerOverflow=on
  Product{,1..4} (5 alike) : Product  OutDataType=sfix(16)  OutScaling=2^0  RndMeth=Zero
  Sum : Sum  Inputs=|-+--  OutDataType=sfix(16)  OutScaling=2^0
  Switch : Switch  Threshold=60  OutDataType=sfix(16)  OutScaling=2^0
  f(es,0) : Constant  Value=16.11  OutDataType=sfix(16)  OutScaling=2^0
  f(es,inf) : Constant  Value=2.1  OutDataType=sfix(16)  OutScaling=2^0
  f(es,max) : Constant  Value=60  OutDataType=sfix(16)  OutScaling=2^0
  k(es) : Constant  Value=0.0675  OutDataType=sfix(16)  OutScaling=2^0
  theta(sp) : Constant  Value=-0.68  OutDataType=sfix(16)  OutScaling=2^0
  w(b,sp) : Constant  OutDataType=sfix(16)  OutScaling=2^0
  w(c,sp) : Constant  Value=5  OutDataType=sfix(16)  OutScaling=2^0
  w(p,sp) : Constant  Value=0.34  OutDataType=sfix(16)  OutScaling=2^0
  f(sp) : Outport  OutDataType=sfix(16)  OutScaling=2^0
  wires:
  w(b,sp)/1 -> Product/2
  f(ab)/1 -> Product/1
  f(ac)/1 -> Product1/1
  w(c,sp)/1 -> Product1/2
  f(ap)/1 -> Product2/1
  w(p,sp)/1 -> Product2/2
  Product/1 -> Sum/1
  Product1/1 -> Sum/2
  Product2/1 -> Sum/3
  theta(sp)/1 -> Sum/4
  Sum/1 -> Product3/1
  k(es)/1 -> Product3/2
  Product3/1 -> Math Function/1
  f(es,inf)/1 -> Add/1, Add1/1
  f(es,0)/1 -> Add/2
  Add/1 -> Product4/1
  Math Function/1 -> Product4/2
  Product4/1 -> Add1/2
  Add1/1 -> Switch/2, Switch/3
  Switch/1 -> f(sp)/1
  f(es,max)/1 -> Switch/1

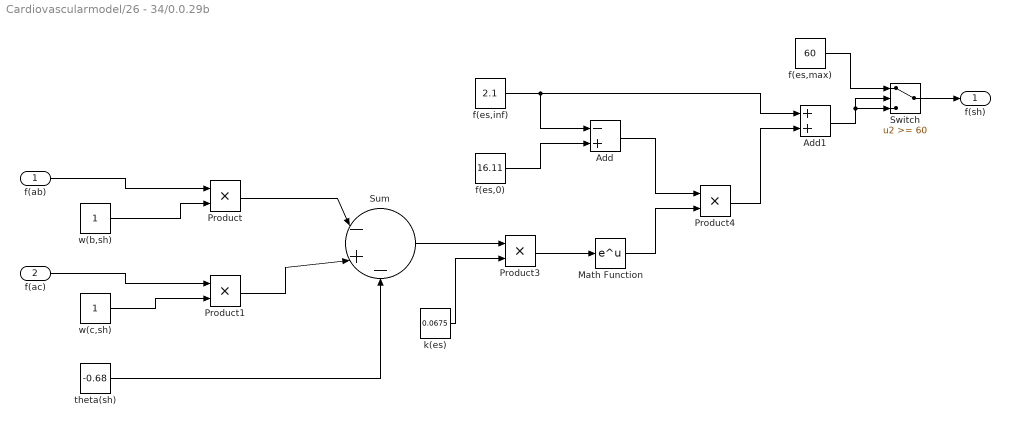
== system Cardiovascularmodel/26 - 34/0.0.29b ==
  f(ab) : Inport  OutDataType=sfix(16)  OutScaling=2^0
  f(ac) : Inport  Port=2  OutDataType=sfix(16)  OutScaling=2^0
  Add : Sum  Inputs=-+  OutDataType=sfix(16)  OutScaling=2^-10
  Add1 : Sum  OutDataType=sfix(16)  OutScaling=2^-10
  Math Function : Math  OutDataType=sfix(16)  OutScaling=2^0  SaturateOnIntegerOverflow=on
  Product{,1,3..4} (4 alike) : Product  OutDataType=sfix(16)  OutScaling=2^0  RndMeth=Zero
  Sum : Sum  Inputs=|-+-  OutDataType=sfix(16)  OutScaling=2^0
  Switch : Switch  Threshold=60  OutDataType=sfix(16)  OutScaling=2^0
  f(es,0) : Constant  Value=16.11  OutDataType=sfix(16)  OutScaling=2^0
  f(es,inf) : Constant  Value=2.1  OutDataType=sfix(16)  OutScaling=2^0
  f(es,max) : Constant  Value=60  OutDataType=sfix(16)  OutScaling=2^0
  k(es) : Constant  Value=0.0675  OutDataType=sfix(16)  OutScaling=2^0
  theta(sh) : Constant  Value=-0.68  OutDataType=sfix(16)  OutScaling=2^0
  w(b,sh) : Constant  OutDataType=sfix(16)  OutScaling=2^0
  w(c,sh) : Constant  OutDataType=sfix(16)  OutScaling=2^0
  f(sh) : Outport  OutDataType=sfix(16)  OutScaling=2^0
  wires:
  w(b,sh)/1 -> Product/2
  f(ab)/1 -> Product/1
  f(ac)/1 -> Product1/1
  w(c,sh)/1 -> Product1/2
  Product/1 -> Sum/1
  Product1/1 -> Sum/2
  theta(sh)/1 -> Sum/3
  Sum/1 -> Product3/1
  k(es)/1 -> Product3/2
  Product3/1 -> Math Function/1
  f(es,inf)/1 -> Add/1, Add1/1
  f(es,0)/1 -> Add/2
  Add/1 -> Product4/1
  Math Function/1 -> Product4/2
  Product4/1 -> Add1/2
  Add1/1 -> Switch/2, Switch/3
  Switch/1 -> f(sh)/1
  f(es,max)/1 -> Switch/1

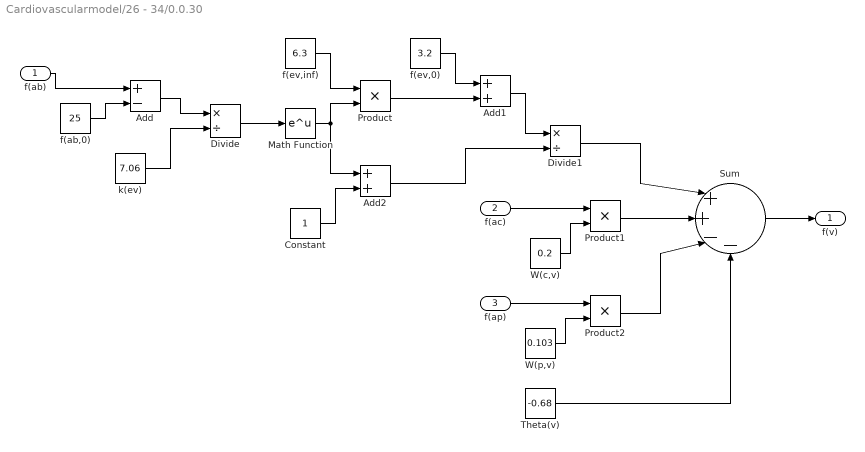
== system Cardiovascularmodel/26 - 34/0.0.30 ==
  f(ab) : Inport  OutDataType=sfix(16)  OutScaling=2^0
  f(ac) : Inport  Port=2  OutDataType=sfix(16)  OutScaling=2^0
  f(ap) : Inport  Port=3  OutDataType=sfix(16)  OutScaling=2^0
  Add : Sum  Inputs=+-  OutDataType=sfix(16)  OutScaling=2^-10
  Add1 : Sum  OutDataType=sfix(16)  OutScaling=2^-10
  Add2 : Sum  OutDataType=sfix(16)  OutScaling=2^-10
  Constant : Constant  OutDataType=sfix(16)  OutScaling=2^0
  Divide : Product  Inputs=*/  OutDataType=sfix(16)  OutScaling=2^-10
  Divide1 : Product  Inputs=*/  OutDataType=sfix(16)  OutScaling=2^-10
  Math Function : Math  OutDataType=sfix(16)  OutScaling=2^0  SaturateOnIntegerOverflow=on
  Product : Product  OutDataType=sfix(16)  OutScaling=2^0  RndMeth=Zero
  Product1 : Product  OutDataType=sfix(16)  OutScaling=2^0  RndMeth=Zero
  Product2 : Product  OutDataType=sfix(16)  OutScaling=2^0  RndMeth=Zero
  Sum : Sum  Inputs=|++--  OutDataType=sfix(16)  OutScaling=2^0
  Theta(v) : Constant  Value=-0.68  OutDataType=sfix(16)  OutScaling=2^0
  W(c,v) : Constant  Value=0.2  OutDataType=sfix(16)  OutScaling=2^0
  W(p,v) : Constant  Value=0.103  OutDataType=sfix(16)  OutScaling=2^0
  f(ab,0) : Constant  Value=25  OutDataType=sfix(16)  OutScaling=2^0
  f(ev,0) : Constant  Value=3.2  OutDataType=sfix(16)  OutScaling=2^0
  f(ev,inf) : Constant  Value=6.3  OutDataType=sfix(16)  OutScaling=2^0
  k(ev) : Constant  Value=7.06  OutDataType=sfix(16)  OutScaling=2^0
  f(v) : Outport  OutDataType=sfix(16)  OutScaling=2^0
  wires:
  f(ab)/1 -> Add/1
  f(ab,0)/1 -> Add/2
  Add/1 -> Divide/1
  k(ev)/1 -> Divide/2
  Divide/1 -> Math Function/1
  f(ev,inf)/1 -> Product/1
  Math Function/1 -> Product/2, Add2/1
  Product/1 -> Add1/2
  f(ev,0)/1 -> Add1/1
  Constant/1 -> Add2/2
  Add1/1 -> Divide1/1
  Add2/1 -> Divide1/2
  f(ac)/1 -> Product1/1
  f(ap)/1 -> Product2/1
  Divide1/1 -> Sum/1
  Product1/1 -> Sum/2
  Product2/1 -> Sum/3
  Theta(v)/1 -> Sum/4
  Sum/1 -> f(v)/1
  W(c,v)/1 -> Product1/2
  W(p,v)/1 -> Product2/2

== system Cardiovascularmodel/26 - 34/0.0.31a ==
  fsp : Inport  OutDataType=sfix(16)  OutScaling=2^0
  0 : Constant  Value=0  OutDataType=sfix(16)  OutScaling=2^0
  1 : Constant  OutDataType=sfix(16)  OutScaling=2^0
  Add1 : Sum  Inputs=++-  OutDataType=sfix(16)  OutScaling=2^-10
  D(R(sp)) : Constant  Value=2  OutDataType=sfix(16)  OutScaling=2^0
  G(R(sp)) : Constant  Value=0.695  OutDataType=sfix(16)  OutScaling=2^0
  Math Function : Math  Operator=log  OutDataType=sfix(16)  OutScaling=2^0  SaturateOnIntegerOverflow=on
  Product : Product  OutDataType=sfix(16)  OutScaling=2^0  RndMeth=Zero
  Switch : Switch  Threshold=2.66  OutDataType=sfix(16)  OutScaling=2^0
  Variable Time Delay : VariableTransportDelay  MaximumDelay=10
  f(es,min) : Constant  Value=2.66  OutDataType=sfix(16)  OutScaling=2^0
  Sigma R sp : Outport  OutDataType=sfix(16)  OutScaling=2^0
  wires:
  fsp/1 -> Switch/2, Variable Time Delay/1
  Math Function/1 -> Product/1
  G(R(sp))/1 -> Product/2
  Product/1 -> Switch/1
  0/1 -> Switch/3
  Switch/1 -> Sigma R sp/1
  Add1/1 -> Math Function/1
  1/1 -> Add1/2
  f(es,min)/1 -> Add1/3
  Variable Time Delay/1 -> Add1/1
  D(R(sp))/1 -> Variable Time Delay/2

== system Cardiovascularmodel/26 - 34/0.0.31c ==
  Delta R(sp) : Inport  OutDataType=sfix(16)  OutScaling=2^0
  Add : Sum  OutDataType=sfix(16)  OutScaling=2^-10
  R(sp0) : Constant  Value=2.49  OutDataType=sfix(16)  OutScaling=2^0
  Rsp : Outport  OutDataType=sfix(16)  OutScaling=2^0
  wires:
  Add/1 -> Rsp/1
  Delta R(sp)/1 -> Add/1
  R(sp0)/1 -> Add/2

== system Cardiovascularmodel/26 - 34/0.0.31d ==
  fsp : Inport  OutDataType=sfix(16)  OutScaling=2^0
  0 : Constant  Value=0  OutDataType=sfix(16)  OutScaling=2^0
  1 : Constant  OutDataType=sfix(16)  OutScaling=2^0
  Add1 : Sum  Inputs=++-  OutDataType=sfix(16)  OutScaling=2^-10
  D(R(mp)) : Constant  Value=2  OutDataType=sfix(16)  OutScaling=2^0
  G(R(mp)) : Constant  Value=2.47  OutDataType=sfix(16)  OutScaling=2^0
  Math Function : Math  Operator=log  OutDataType=sfix(16)  OutScaling=2^0  SaturateOnIntegerOverflow=on
  Product : Product  OutDataType=sfix(16)  OutScaling=2^0  RndMeth=Zero
  Switch : Switch  Threshold=2.66  OutDataType=sfix(16)  OutScaling=2^0
  Variable Time Delay : VariableTransportDelay  MaximumDelay=10
  f(es,min) : Constant  Value=2.66  OutDataType=sfix(16)  OutScaling=2^0
  Sigma R mp : Outport  OutDataType=sfix(16)  OutScaling=2^0
  wires:
  fsp/1 -> Switch/2, Variable Time Delay/1
  Math Function/1 -> Product/1
  G(R(mp))/1 -> Product/2
  Product/1 -> Switch/1
  0/1 -> Switch/3
  Switch/1 -> Sigma R mp/1
  Add1/1 -> Math Function/1
  Variable Time Delay/1 -> Add1/1
  1/1 -> Add1/2
  f(es,min)/1 -> Add1/3
  D(R(mp))/1 -> Variable Time Delay/2

== system Cardiovascularmodel/26 - 34/0.0.31f ==
  Delta R(mp) : Inport  OutDataType=sfix(16)  OutScaling=2^0
  Add : Sum  OutDataType=sfix(16)  OutScaling=2^-10
  R(sp0) : Constant  Value=2.106  OutDataType=sfix(16)  OutScaling=2^0
  Rmp : Outport  OutDataType=sfix(16)  OutScaling=2^0
  wires:
  Add/1 -> Rmp/1
  Delta R(mp)/1 -> Add/1
  R(sp0)/1 -> Add/2

== system Cardiovascularmodel/26 - 34/0.0.31g ==
  fsp : Inport  OutDataType=sfix(16)  OutScaling=2^0
  0 : Constant  Value=0  OutDataType=sfix(16)  OutScaling=2^0
  1 : Constant  OutDataType=sfix(16)  OutScaling=2^0
  Add1 : Sum  Inputs=++-  OutDataType=sfix(16)  OutScaling=2^-10
  D(R(ep)) : Constant  Value=2  OutDataType=sfix(16)  OutScaling=2^0
  G(R(ep)) : Constant  Value=1.94  OutDataType=sfix(16)  OutScaling=2^0
  Math Function : Math  Operator=log  OutDataType=sfix(16)  OutScaling=2^0  SaturateOnIntegerOverflow=on
  Product : Product  OutDataType=sfix(16)  OutScaling=2^0  RndMeth=Zero
  Switch : Switch  Threshold=2.66  OutDataType=sfix(16)  OutScaling=2^0
  Variable Time Delay : VariableTransportDelay  MaximumDelay=10
  f(es,min) : Constant  Value=2.66  OutDataType=sfix(16)  OutScaling=2^0
  Sigma R ep : Outport  OutDataType=sfix(16)  OutScaling=2^0
  wires:
  D(R(ep))/1 -> Variable Time Delay/2
  fsp/1 -> Switch/2, Variable Time Delay/1
  Math Function/1 -> Product/1
  G(R(ep))/1 -> Product/2
  Product/1 -> Switch/1
  0/1 -> Switch/3
  Switch/1 -> Sigma R ep/1
  Variable Time Delay/1 -> Add1/1
  Add1/1 -> Math Function/1
  1/1 -> Add1/2
  f(es,min)/1 -> Add1/3

== system Cardiovascularmodel/26 - 34/0.0.31i ==
  Delta R(mp) : Inport  OutDataType=sfix(16)  OutScaling=2^0
  Add : Sum  OutDataType=sfix(16)  OutScaling=2^-10
  R(sp0) : Constant  Value=1.655  OutDataType=sfix(16)  OutScaling=2^0
  Rep : Outport  OutDataType=sfix(16)  OutScaling=2^0
  wires:
  Add/1 -> Rep/1
  Delta R(mp)/1 -> Add/1
  R(sp0)/1 -> Add/2

== system Cardiovascularmodel/26 - 34/0.0.32a ==
  fsh : Inport  OutDataType=fixdt(1, 16)  OutScaling=2^0
  Constant : Constant  Value=0  OutDataType=fixdt(1, 16)  OutScaling=2^0
  Constant1 : Constant  OutDataType=fixdt(1, 16)  OutScaling=2^0
  D(Emax,rv) : Constant  Value=2  OutDataType=fixdt(1, 16)  OutScaling=2^0
  G(Emax,rv) : Constant  Value=0.282  OutDataType=fixdt(1, 16)  OutScaling=2^0
  Math Function : Math  Operator=log  OutDataType=fixdt(1, 16)  OutScaling=2^0  SaturateOnIntegerOverflow=on
  Product : Product  OutDataType=fixdt(1, 16)  OutScaling=2^0  RndMeth=Zero
  Subtract1 : Sum  Inputs=++-  OutDataType=fixdt(1, 16)  OutScaling=2^-10
  Switch : Switch  Threshold=2.66  OutDataType=fixdt(1, 16)  OutScaling=2^0
  Variable Time Delay : VariableTransportDelay  MaximumDelay=10
  f(es,min) : Constant  Value=2.66  OutDataType=fixdt(1, 16)  OutScaling=2^0
  sigma(Emax,rv) : Outport  OutDataType=fixdt(1, 16)  OutScaling=2^0
  wires:
  fsh/1 -> Switch/2, Variable Time Delay/1
  Switch/1 -> sigma(Emax,rv)/1
  Constant/1 -> Switch/3
  G(Emax,rv)/1 -> Product/1
  Product/1 -> Switch/1
  f(es,min)/1 -> Subtract1/3
  Constant1/1 -> Subtract1/1
  Subtract1/1 -> Math Function/1
  Math Function/1 -> Product/2
  Variable Time Delay/1 -> Subtract1/2
  D(Emax,rv)/1 -> Variable Time Delay/2

== system Cardiovascularmodel/26 - 34/0.0.32f ==
  fsh : Inport  OutDataType=fixdt(1, 16)  OutScaling=2^0
  Constant : Constant  Value=0  OutDataType=fixdt(1, 16)  OutScaling=2^0
  Constant1 : Constant  OutDataType=fixdt(1, 16)  OutScaling=2^0
  D(Emax,lv) : Constant  Value=2  OutDataType=fixdt(1, 16)  OutScaling=2^0
  G(Emax,lv) : Constant  Value=0.475  OutDataType=fixdt(1, 16)  OutScaling=2^0
  Math Function : Math  Operator=log  OutDataType=fixdt(1, 16)  OutScaling=2^0  SaturateOnIntegerOverflow=on
  Product : Product  OutDataType=fixdt(1, 16)  OutScaling=2^0  RndMeth=Zero
  Subtract1 : Sum  Inputs=++-  OutDataType=fixdt(1, 16)  OutScaling=2^-10
  Switch : Switch  Threshold=2.66  OutDataType=fixdt(1, 16)  OutScaling=2^0
  Variable Time Delay : VariableTransportDelay  MaximumDelay=10
  f(es,min) : Constant  Value=2.66  OutDataType=fixdt(1, 16)  OutScaling=2^0
  sigma(Emax,lv) : Outport  OutDataType=fixdt(1, 16)  OutScaling=2^0
  wires:
  fsh/1 -> Switch/2, Variable Time Delay/1
  Switch/1 -> sigma(Emax,lv)/1
  G(Emax,lv)/1 -> Product/1
  Product/1 -> Switch/1
  Math Function/1 -> Product/2
  f(es,min)/1 -> Subtract1/3
  Variable Time Delay/1 -> Subtract1/2
  Constant1/1 -> Subtract1/1
  Subtract1/1 -> Math Function/1
  Constant/1 -> Switch/3
  D(Emax,lv)/1 -> Variable Time Delay/2

== system Cardiovascularmodel/26 - 34/0.0.33d ==
  fsh : Inport  OutDataType=fixdt(1, 16)  OutScaling=2^0
  Constant : Constant  Value=0  OutDataType=fixdt(1, 16)  OutScaling=2^0
  Constant1 : Constant  OutDataType=fixdt(1, 16)  OutScaling=2^0
  D(Ts) : Constant  Value=2  OutDataType=fixdt(1, 16)  OutScaling=2^0
  G(Ts) : Constant  Value=-0.13  OutDataType=fixdt(1, 16)  OutScaling=2^0
  Math Function : Math  Operator=log  OutDataType=fixdt(1, 16)  OutScaling=2^0  SaturateOnIntegerOverflow=on
  Product : Product  OutDataType=fixdt(1, 16)  OutScaling=2^0  RndMeth=Zero
  Subtract1 : Sum  Inputs=++-  OutDataType=fixdt(1, 16)  OutScaling=2^-10
  Switch : Switch  Threshold=2.66  OutDataType=fixdt(1, 16)  OutScaling=2^0
  Variable Time Delay : VariableTransportDelay  MaximumDelay=10
  f(es,min) : Constant  Value=2.66  OutDataType=fixdt(1, 16)  OutScaling=2^0
  sigma(Ts) : Outport  OutDataType=fixdt(1, 16)  OutScaling=2^0
  wires:
  fsh/1 -> Switch/2, Variable Time Delay/1
  Switch/1 -> sigma(Ts)/1
  Constant/1 -> Switch/3
  G(Ts)/1 -> Product/1
  Product/1 -> Switch/1
  Constant1/1 -> Subtract1/1
  f(es,min)/1 -> Subtract1/3
  Subtract1/1 -> Math Function/1
  Math Function/1 -> Product/2
  Variable Time Delay/1 -> Subtract1/2
  D(Ts)/1 -> Variable Time Delay/2

== system Cardiovascularmodel/26 - 34/0.0.33e ==
  fv : Inport  OutDataType=fixdt(1, 16)  OutScaling=2^0
  D(Tv) : Constant  Value=0.2  OutDataType=fixdt(1, 16)  OutScaling=2^0
  G(Ty) : Constant  Value=-0.09  OutDataType=fixdt(1, 16)  OutScaling=2^0
  Product : Product  OutDataType=fixdt(1, 16)  OutScaling=2^0  RndMeth=Zero
  Variable Time Delay : VariableTransportDelay  MaximumDelay=10
  sigma(Tv) : Outport  OutDataType=fixdt(1, 16)  OutScaling=2^0
  wires:
  G(Ty)/1 -> Product/1
  Product/1 -> sigma(Tv)/1
  Variable Time Delay/1 -> Product/2
  D(Tv)/1 -> Variable Time Delay/2
  fv/1 -> Variable Time Delay/1

== system Cardiovascularmodel/26 - 34/0.0.34c ==
  fsp : Inport  OutDataType=fixdt(1, 16)  OutScaling=2^0
  Constant : Constant  Value=0  OutDataType=fixdt(1, 16)  OutScaling=2^0
  Constant1 : Constant  OutDataType=fixdt(1, 16)  OutScaling=2^0
  D(V(u,mv)) : Constant  Value=5  OutDataType=fixdt(1, 16)  OutScaling=2^0
  G(V(u,mv)) : Constant  Value=-58.29  OutDataType=fixdt(1, 16)  OutScaling=2^0
  Math Function : Math  Operator=log  OutDataType=fixdt(1, 16)  OutScaling=2^0  SaturateOnIntegerOverflow=on
  Product : Product  OutDataType=fixdt(1, 16)  OutScaling=2^0  RndMeth=Zero
  Subtract1 : Sum  Inputs=++-  OutDataType=fixdt(1, 16)  OutScaling=2^-10
  Switch : Switch  Threshold=2.66  OutDataType=fixdt(1, 16)  OutScaling=2^0
  Variable Time Delay : VariableTransportDelay  MaximumDelay=10
  f(es,min) : Constant  Value=2.66  OutDataType=fixdt(1, 16)  OutScaling=2^0
  sigma(V(u,mv)) : Outport  OutDataType=fixdt(1, 16)  OutScaling=2^0
  wires:
  fsp/1 -> Switch/2, Variable Time Delay/1
  Switch/1 -> sigma(V(u,mv))/1
  Constant/1 -> Switch/3
  G(V(u,mv))/1 -> Product/1
  Product/1 -> Switch/1
  Math Function/1 -> Product/2
  Subtract1/1 -> Math Function/1
  f(es,min)/1 -> Subtract1/3
  Constant1/1 -> Subtract1/1
  Variable Time Delay/1 -> Subtract1/2
  D(V(u,mv))/1 -> Variable Time Delay/2

== system Cardiovascularmodel/26 - 34/0.0.34f ==
  fsp : Inport  OutDataType=fixdt(1, 16)  OutScaling=2^0
  Constant : Constant  Value=0  OutDataType=fixdt(1, 16)  OutScaling=2^0
  Constant1 : Constant  OutDataType=fixdt(1, 16)  OutScaling=2^0
  D(V(u,sv)) : Constant  Value=5  OutDataType=fixdt(1, 16)  OutScaling=2^0
  G(V(u,sv)) : Constant  Value=-265.4  OutDataType=fixdt(1, 16)  OutScaling=2^0
  Math Function : Math  Operator=log  OutDataType=fixdt(1, 16)  OutScaling=2^0  SaturateOnIntegerOverflow=on
  Product : Product  OutDataType=fixdt(1, 16)  OutScaling=2^0  RndMeth=Zero
  Subtract1 : Sum  Inputs=++-  OutDataType=fixdt(1, 16)  OutScaling=2^-10
  Switch : Switch  Threshold=2.66  OutDataType=fixdt(1, 16)  OutScaling=2^0
  Variable Time Delay : VariableTransportDelay  MaximumDelay=10
  f(es,min) : Constant  Value=2.66  OutDataType=fixdt(1, 16)  OutScaling=2^0
  sigma(V(u,sv)) : Outport  OutDataType=fixdt(1, 16)  OutScaling=2^0
  wires:
  fsp/1 -> Switch/2, Variable Time Delay/1
  Switch/1 -> sigma(V(u,sv))/1
  Constant/1 -> Switch/3
  G(V(u,sv))/1 -> Product/1
  Product/1 -> Switch/1
  Constant1/1 -> Subtract1/1
  f(es,min)/1 -> Subtract1/3
  Subtract1/1 -> Math Function/1
  Math Function/1 -> Product/2
  Variable Time Delay/1 -> Subtract1/2
  D(V(u,sv))/1 -> Variable Time Delay/2
